simulink model "simulink_esame"  (R2024a)
settings: Solver=VariableStepAuto  StartTime=0.0  StopTime=10.0  RelTol=1e-3
values from neighbouring files (symbols this model uses):
  A = [-1 4;0 -5]    [TE_ES2_2023_01_09.m]    (also in fobj_esame.m)
  alfa = -inv(C*(A-B*K3)*B)    [TE_ES2_2023_01_09.m]    (also in fobj_esame.m = K(1))
  B = [1 1]'    [TE_ES2_2023_01_09.m]    (also in fobj_esame.m)
  C = [1 0]    [TE_ES2_2023_01_09.m]    (also in fobj_esame.m)
  K1 = K(2)    [fobj_esame.m]
  K2 = place(A,B,E2)    [TE_ES2_2023_01_09.m]    (also in fobj_esame.m = K(3))
  y0 = 5    [fobj_esame.m]
settings Model: Creator=stefa  LastModifiedBy=stefa

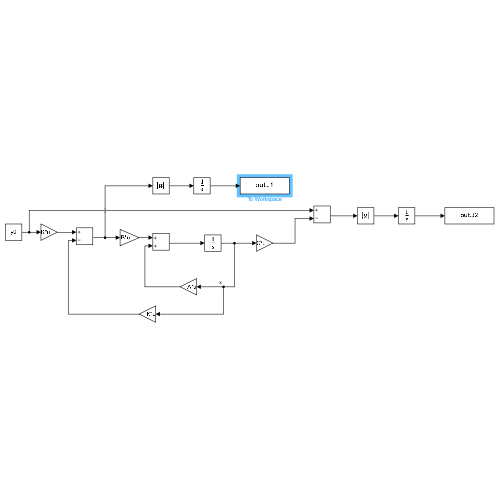
[thumbnail: Simulink's stored preview of the top-level diagram]
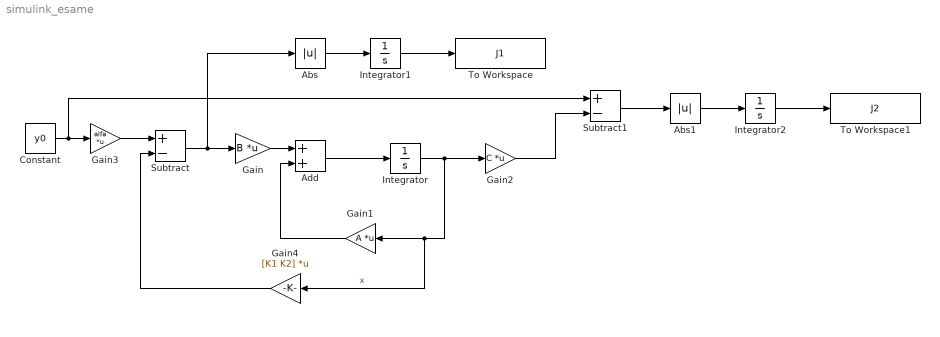
== system simulink_esame ==
  Abs : Abs  SaturateOnIntegerOverflow=off
  Abs1 : Abs  SaturateOnIntegerOverflow=off
  Add : Sum
  Constant : Constant  Value=y0
  Gain : Gain  Gain=B  Multiplication=Matrix(K*u)
  Gain1 : Gain  Gain=A  Multiplication=Matrix(K*u)
  Gain2 : Gain  Gain=C  Multiplication=Matrix(K*u)
  Gain3 : Gain  Gain=alfa  Multiplication=Matrix(K*u)
  Gain4 : Gain  Gain=[K1 K2]  Multiplication=Matrix(K*u)
  Integrator : Integrator
  Integrator1 : Integrator
  Integrator2 : Integrator
  Subtract : Sum  Inputs=+-
  Subtract1 : Sum  Inputs=+-
  To Workspace : ToWorkspace  VariableName=J1  SampleTime=-1
  To Workspace1 : ToWorkspace  VariableName=J2  SampleTime=-1
  wires:
  Gain/1 -> Add/1
  Add/1 -> Integrator/1
  Integrator/1 -> Gain2/1, Gain1/1, Gain4/1  "x"
  Gain1/1 -> Add/2
  Constant/1 -> Subtract1/1, Gain3/1
  Subtract/1 -> Abs/1, Gain/1
  Gain3/1 -> Subtract/1
  Gain4/1 -> Subtract/2
  Abs/1 -> Integrator1/1
  Integrator1/1 -> To Workspace/1
  Gain2/1 -> Subtract1/2
  Abs1/1 -> Integrator2/1
  Integrator2/1 -> To Workspace1/1
  Subtract1/1 -> Abs1/1
